simulink model "model"  (R2020b)
settings: Solver=VariableStepAuto  StartTime=0.0  StopTime=10.0  RelTol=1e-3
settings Model: Creator=Pavan  LastModifiedBy=Pavan

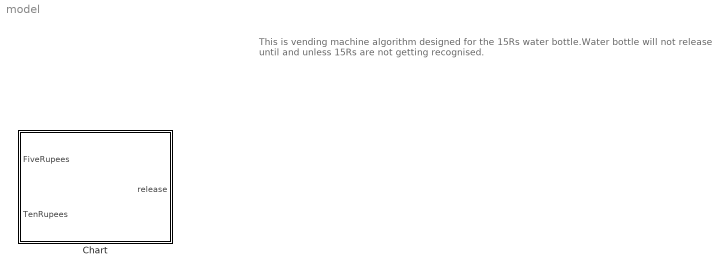
== system model ==
  note: This is vending machine algorithm designed for the 15Rs water bottle.Water bottle will not release until and unless 15Rs are not getting recognised.
  Chart : Stateflow chart  TreatAsAtomicUnit=on

== stateflow chart model/Chart ==
  state Zero
  state TenRupeesCoin
  state return
  state fiveRupeescoin
  TenRupeesCoin -> return [order 2] : after(3,sec){release=0}
  Zero -> TenRupeesCoin [order 2] : [TenRupees==1]{release=0}
  (default) -> Zero
  return -> Zero : after(1,sec){release=0}
  TenRupeesCoin -> Zero [order 1] : [FiveRupees==1]{release=1}
  fiveRupeescoin -> TenRupeesCoin [order 2] : [FiveRupees==1]{release=0}
  fiveRupeescoin -> return [order 3] : after(3,sec){release=0}
  fiveRupeescoin -> Zero [order 1] : [TenRupees==1]{release=1}
  Zero -> fiveRupeescoin [order 1] : [FiveRupees==1]{release=0}
  data: FiveRupees input; TenRupees input; release output
